simulink model "Complete_Model"  (R2018b)
settings: Solver=VariableStepAuto  StartTime=0.0  StopTime=200  RelTol=1e-3
values from neighbouring files (symbols this model uses):
  alpha = 0.5736    [constants.m]
  c_damp = 0.00495    [constants.m]
  delay = 0.8    [constants.m]
  dis_torque = 0.001    [constants.m]
  in_nu = 0.0001    [constants.m]
  J_r = 0.0004    [constants.m]
  J_s = 31.38    [constants.m]
  noise = 10^-9    (= 1e-09)    [constants.m]
  T_sat = 0.05    [constants.m]
  time_cons = 0.5    [constants.m]
  w_mode = 2.6268    [constants.m]
  w_sat = 2800*2*pi/60    (= 293.215314335)    [constants.m]
undefined symbols (not defined in the file or in its folder): sigbuilder_block
settings Model: Creator=Yavuz  LastModifiedBy=Yavuz

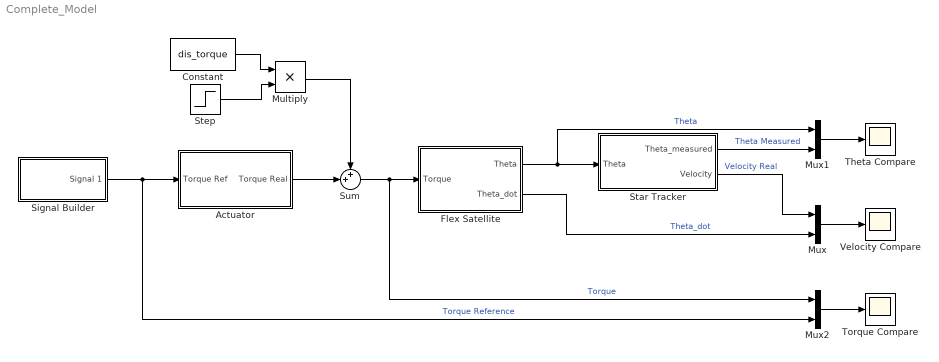
== system Complete_Model ==
  Actuator : Subsystem
  Constant : Constant  Value=dis_torque
  Flex Satellite : Subsystem
  Multiply : Product
  Mux : Mux  Inputs=2
  Mux1 : Mux  Inputs=2
  Mux2 : Mux  Inputs=2
  Signal Builder : Subsystem  Tag=STV Subsys  LoadFcn=sigbuilder_block('load');  StartFcn=sigbuilder_block('start');  StopFcn=sigbuilder_block('stop');  ClipboardFcn=sigbuilder_block('clipboard');  mask(Sigbuilder block){tuvar=[0:10]}
      mask help: Simulink:masks:SigbuilderBlock_MD
      mask init:
      | if ~strcmp(get_param(bdroot(gcbh),'SimulationStatus'),'stopped') tuvar = sigbuilder_block('maskInit'); end
      settings: CopyFcn=sigbuilder_block('copy');  DeleteFcn=sigbuilder_block('delete');  ModelCloseFcn=sigbuilder_block('modelClose');  PreSaveFcn=sigbuilder_block('preSave');  PauseFcn=sigbuilder_block('pause');  ContinueFcn=sigbuilder_block('continue');  NameChangeFcn=sigbuilder_block('namechange');  OpenFcn=sigbuilder_block('open',[6 30 1428 681.75 ]);  CloseFcn=sigbuilder_block('close');
      mask Display: plot(0, 0, 100, 100,[2, 2, 32, 32, 2], [68, 8, 8, 68, 68],[32, 2], [38, 38], [32, 19, 2],[53, 60, 44], [32, 17, 17, 2],[16, 16, 31, 31]);txt = getActiveGroup(gcbh);text(2, 100, txt,'verticalAlignment', 'top');
  Star Tracker : Subsystem
  Step : Step  Time=100  SampleTime=0
  Sum : Sum  Inputs=++|
  Theta Compare : Scope
  Torque Compare : Scope
  Velocity Compare : Scope
  wires:
  Flex Satellite/1(Theta) -> Mux1/1, Star Tracker/1(Theta)  "Theta"
  Sum/1 -> Mux2/1, Flex Satellite/1(Torque)  "Torque"
  Actuator/1(Torque Real) -> Sum/2
  Constant/1 -> Multiply/1
  Step/1 -> Multiply/2
  Multiply/1 -> Sum/1
  Star Tracker/2(Velocity) -> Mux/1  "Velocity Real"
  Flex Satellite/2(Theta_dot) -> Mux/2  "Theta_dot"
  Mux/1 -> Velocity Compare/1
  Mux1/1 -> Theta Compare/1
  Star Tracker/1(Theta_measured) -> Mux1/2  "Theta Measured"
  Mux2/1 -> Torque Compare/1
  Signal Builder/1(Signal 1) -> Mux2/2, Actuator/1(Torque Ref)  "Torque Reference"

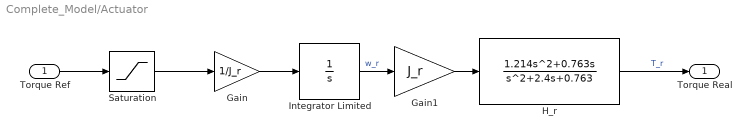
== system Complete_Model/Actuator ==
  Torque Ref : Inport
  Gain : Gain  Gain=1/J_r
  Gain1 : Gain  Gain=J_r
  H_r : TransferFcn  Numerator=[1.214 0.763 0]  Denominator=[1 2.4 0.763]
  Integrator Limited : Integrator  LimitOutput=on  UpperSaturationLimit=w_sat  LowerSaturationLimit=0
  Saturation : Saturate  UpperLimit=T_sat  LowerLimit=-T_sat
  Torque Real : Outport
  wires:
  Saturation/1 -> Gain/1
  Torque Ref/1 -> Saturation/1
  Gain1/1 -> H_r/1
  Gain/1 -> Integrator Limited/1
  H_r/1 -> Torque Real/1  "T_r"
  Integrator Limited/1 -> Gain1/1  "w_r"

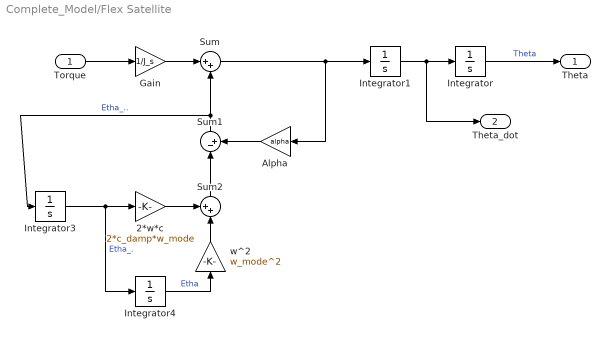
== system Complete_Model/Flex Satellite ==
  Torque : Inport
  2*w*c : Gain  Gain=2*c_damp*w_mode
  Alpha : Gain  Gain=alpha
  Gain : Gain  Gain=1/J_s
  Integrator : Integrator
  Integrator1 : Integrator
  Integrator3 : Integrator
  Integrator4 : Integrator  InitialCondition=in_nu
  Sum : Sum  Inputs=|++
  Sum1 : Sum  Inputs=|-+
  Sum2 : Sum  Inputs=++|
  w^2 : Gain  Gain=w_mode^2
  Theta : Outport
  Theta_dot : Outport  Port=2
  wires:
  Sum/1 -> Integrator1/1, Alpha/1
  Sum1/1 -> Integrator3/1, Sum/2  "Etha_.."
  Gain/1 -> Sum/1
  Integrator1/1 -> Theta_dot/1, Integrator/1
  Integrator3/1 -> Integrator4/1, 2*w*c/1  "Etha_."
  Sum2/1 -> Sum1/1
  Torque/1 -> Gain/1
  2*w*c/1 -> Sum2/1
  Integrator/1 -> Theta/1  "Theta"
  w^2/1 -> Sum2/2
  Integrator4/1 -> w^2/1  "Etha"
  Alpha/1 -> Sum1/2

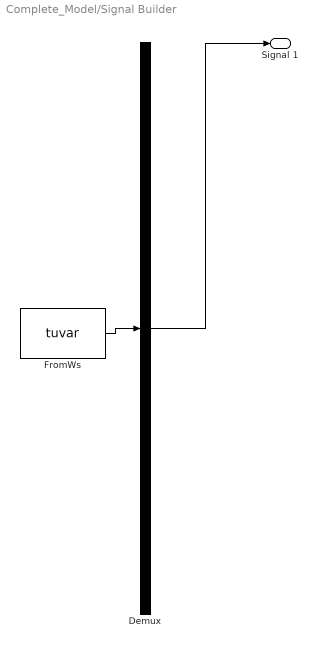
== system Complete_Model/Signal Builder ==
  Demux : Demux  Tag=STV Demux  Outputs=1
  FromWs : FromWorkspace  Tag=STV FromWs  VariableName=tuvar  SampleTime=0
      SigBuilderData=|
      | common.afterFinalStr = 'Extrapolate'
      | common.sampleTime = 0
      | dataSet.timeRange = [0 200]
      | dataSet.name = 'Group 1'
      | sbobj.Groups.Name = 'Group 1'
      | sbobj.Groups.Signals.Name = 'Signal 1'
      | sbobj.Groups.Signals.XData = [0 20 20 80 80 140 140 200]
      | sbobj.Groups.Signals.YData = [0 0 0.003 0.003 -0.003 -0.003 0 0]
      | sbobj.Groups.TimeRange = [0 200]
  Signal 1 : Outport  Tag=STV Outport
  wires:
  Demux/1 -> Signal 1/1
  FromWs/1 -> Demux/1

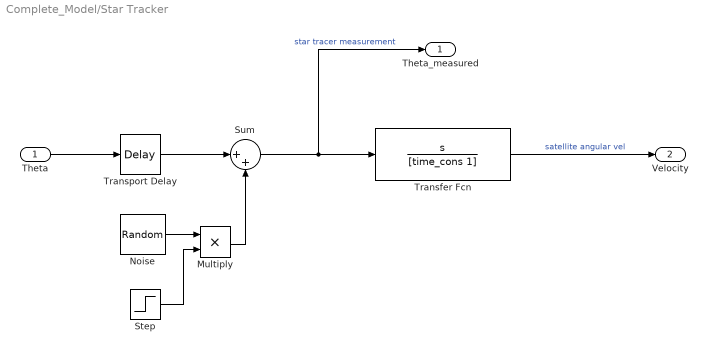
== system Complete_Model/Star Tracker ==
  Theta : Inport
  Multiply : Product
  Noise : RandomNumber  Variance=noise  SampleTime=0.1
  Step : Step  Time=160  SampleTime=0
  Sum : Sum  Inputs=|++
  Transfer Fcn : TransferFcn  Numerator=[1 0]  Denominator=[time_cons 1]
  Transport Delay : TransportDelay  DelayTime=delay
  Theta_measured : Outport
  Velocity : Outport  Port=2
  wires:
  Theta/1 -> Transport Delay/1
  Sum/1 -> Theta_measured/1, Transfer Fcn/1  "star tracer measurement"
  Transport Delay/1 -> Sum/1
  Transfer Fcn/1 -> Velocity/1  "satellite angular vel"
  Noise/1 -> Multiply/1
  Step/1 -> Multiply/2
  Multiply/1 -> Sum/2
